simulink model "asbQuadcopters_SiFi"  (Simulink 9.1)
settings: Solver=VariableStepAuto  StartTime=0.0  StopTime=TFinal  RelTol=1e-3
values from neighbouring files (symbols this model uses):
  Controller =     [data_set.mat]
  Estimator =     [data_set.mat]
  g = 9.81    [data_set.mat]
  init =     [data_set.mat]
  rho = 1.184    [data_set.mat]
  sensorCalibrationData = [0.09 -0.06 -9.473 -0.0095 -0.0075 0.0015 101270.95 0.2]    [data_set.mat]
  Sensors =     [data_set.mat]
  States =     [data_set.mat]
  takeOffDuration = 1    [data_set.mat]
  Ts = 0.005    [data_set.mat]
  Vehicle =     [data_set.mat]
undefined symbols (not defined in the file or in its folder): DiscIntNeverNeededParam, Discrete, Earth, ft, m, s, sigbuilder_block, Time, WGS84
libraries: F_Line_block x565, simulink x39, aerolibconvert2 x4, sharedutil x3, ctrlSharedLib x3, sharedtransform x3, shared6dof x1, aerolibasang x1, aerolibtransform2 x1, aerolibnav x1, aerolibanimutils x1
(part 1 of 4)
settings Model: SuppressorTable="22 serialization::archive 11 0 6 0 0 1 8 0 0 0 0 6 0 0 1 0 44 asbQuadcopters_SiFi/Command/Live Time  Ticks 0 6 0 0 2 8 0 0 0 0 6 40 SimulinkFixedPoint:util:Overflowoccurred 0 0 0 6 0  0  0 0 0 0 8 20160523 0 0 0 10 57 55 0 1 41 Simulink:DataType:WarningOverFlowDetected 0 0 0  0  8 20160523 0 10 57 55 0 1"  LogicAnalyzerSignalOrdering=2e0c0a72-345e-4dc5-9c0e-29032ec30a1e,a96d9f9d-3ef5-4050-b6b8-b8019fd01667,c8d366ad-4d1f-40bd-a54a-09e26b883270,8941bdc4-4fa0-4569-8040-854ce7cb60c2,e7686d44-45c9-4c55-ba5d-06b91bc522a8,a75aae3c-0a7a-4dbc-8a75-97ed30805da8,7c481f21-a942-450d-9b23-3950506eae04,f4ffd508-2ff6-4be3-84ec-4b50dbf29143,1f3924a1-458c-46a2-8b2c-9c14621b8789,e4a67875-028c-4c14-9c8e-409b915de7ac,3b040215-8b3b-4fa4-83ba-2b8f885f07c0,7ff985bf-1692-4a42-b522-9402795b0a0a,96801311-fbc9-43fc-990a-89459d04cf60,3f7e7f5b-3af5-4c93-b146-0b101a8142d3,0d3d2d37-5424-425c-a4de-334d08617026,580b7cd5-bf48-4c17-856d-375ec7fff404,90f02cb4-483b-4429-aad1-b2fbf7021789,01f89b71-6786-463e-ad11-352fa7f1c28f,02989868-8137-4d3a-8960-166047eeff4b,308ffb0e-b64a-44ed-9876-4b581e92a88e,997ea37c-b9fb-41ea-9c95-cc50f5cdec72,ae01c4b6-24f8-47f4-a500-9399ba671a3d,bf52121c-d275-4d5a-9ed0-41089465bc65  Creator=DES  LastModifiedBy=dongw
settings DataIOCC: SaveFormat=Dataset
settings OptimizationCC: LifeSpan=auto
settings DebuggingCC: UnderspecifiedInitializationDetection=Simplified  MergeDetectMultiDrivingBlocksExec=error  SFUnexpectedBacktrackingDiag=error  SFNoUnconditionalDefaultTransitionDiag=error  SFExecutionAtInitializationDiag=warning
settings HardwareCC: ProdBitPerPointer=64  ProdBitPerSizeT=64  ProdBitPerPtrDiffT=64  ProdLargestAtomicFloat=Float  ProdIntDivRoundTo=Zero  ProdEndianess=LittleEndian  ProdWordSize=64  ProdHWDeviceType=Intel->x86-64 (Windows64)
settings ModelReferenceCC: PropagateSignalLabelsOutOfModel=on
settings CodeAppCC: StateflowObjectComments=off
settings GRTTargetCC: TargetLangStandard=C99 (ISO)  CombineOutputUpdateFcns=on  GRTInterface=off
settings ConfigComp: CovMetricSettings=dwe  CovHtmlReporting=off  CovSaveCumulativeToWorkspaceVar=off  CovSaveSingleToWorkspaceVar=off  CovExternalEMLEnable=on

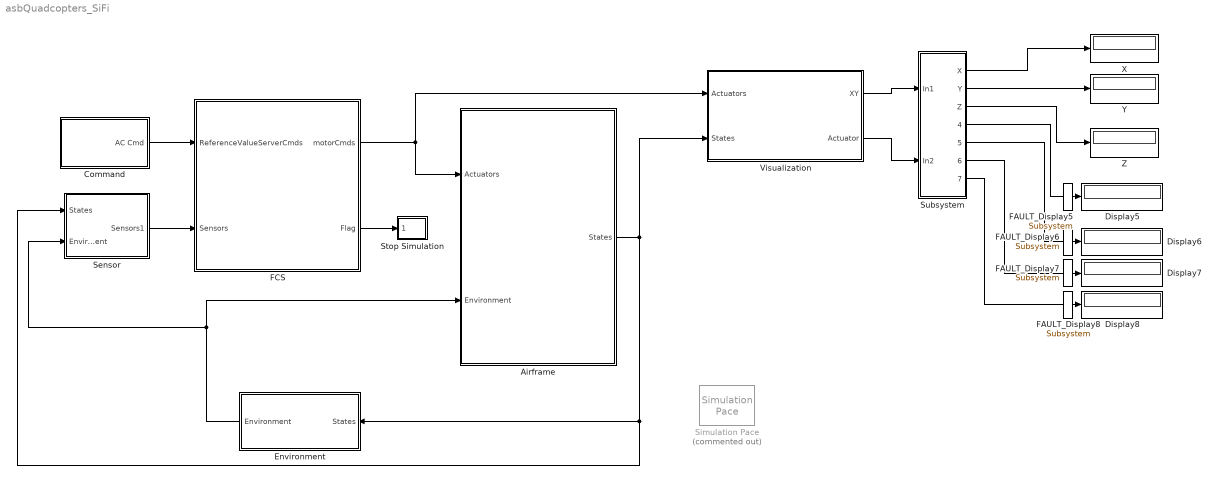
== system asbQuadcopters_SiFi ==
  Airframe : Subsystem  TreatAsAtomicUnit=on
  Command : Subsystem
  Display{5..8} (4 alike) : Display
  FAULT_Display{5..8} (4 alike) : F_Line_block/Subsystem
  Environment : Subsystem
  FCS : Subsystem
  Sensor : Subsystem
  Simulation Pace : aerolibanimutils/Simulation Pace  Commented=on  SimulationPace=1  SleepMode=MATLAB Thread  OutputPaceError=off  SampleTime=Ts
      settings: AttributesFormatString=%<SimulationPace> sec/sec
  Stop Simulation : Subsystem
  Subsystem : Subsystem
  Visualization : Subsystem
  X : Display
  Y : Display
  Z : Display
  wires:
  Command/1(AC Cmd) -> FCS/1(ReferenceValueServerCmds)
  Sensor/1(Sensors1) -> FCS/2(Sensors)
  Airframe/1(States) -> Visualization/2(States), Sensor/1(States), Environment/1(States)
  Environment/1(Environment) -> Sensor/2(Environment), Airframe/2(Environment)
  FCS/2(Flag) -> Stop Simulation/1(Flags)
  FCS/1(motorCmds) -> Visualization/1(Actuators), Airframe/1(Actuators)
  Visualization/1(XY) -> Subsystem/1(In1)
  Visualization/2(Actuator) -> Subsystem/2(In2)
  Subsystem/1(X) -> X/1
  Subsystem/2(Y) -> Y/1
  Subsystem/3(Z) -> Z/1
  Subsystem/4(Motor 1) -> Display5/1
  Subsystem/5(Motor 2) -> Display6/1
  Subsystem/6(Motor 3) -> Display7/1
  Subsystem/7(Motor 4) -> Display8/1

== system asbQuadcopters_SiFi/Airframe ==
  Actuators : Inport
  Environment : Inport  Port=2
  6DOF (Quaternion) : shared6dof/6DOF (Euler Angles)  units=Metric (MKS)  mtype=Fixed  rep=Euler Angles  xme_0=init.posNED  Vm_0=init.vb  eul_0=init.euler  pm_0=init.angRates  mass_0=Vehicle.Airframe.mass  mass_e=0.5  mass_f=2.0  inertia=Vehicle.Airframe.inertia  inertia_e=eye(3)  inertia_f=2*eye(3)  k_quat=Vehicle.SixDOF.quatGain  vre_flag=on  abi_flag=on  aMode=aMode
      settings: SourceProductBaseCode=AE
  FAULT_6DOF (Quaternion) : F_Line_block/Subsystem
  FAULT_6DOF (Quaternion)_2 : F_Line_block/Subsystem
  AC model : Subsystem
  Bus setup : Subsystem
  Position on Earth : Subsystem  Priority=1  TreatAsAtomicUnit=on
  Terminator : Terminator
  FAULT_Terminator : F_Line_block/Subsystem
  States : Outport
  FAULT_States : F_Line_block/Subsystem
  wires:
  Actuators/1 -> AC model/1(Actuators)
  Environment/1 -> AC model/2(Environment)
  AC model/1(F_cg) -> FAULT_6DOF (Quaternion)/1
  FAULT_6DOF (Quaternion)/1 -> 6DOF (Quaternion)/1
  AC model/2(M_cg) -> FAULT_6DOF (Quaternion)_2/1
  FAULT_6DOF (Quaternion)_2/1 -> 6DOF (Quaternion)/2
  6DOF (Quaternion)/1 -> Bus setup/2(V_ned)
  6DOF (Quaternion)/2 -> Position on Earth/1(Xe), Bus setup/3(X_ned)
  6DOF (Quaternion)/3 -> Bus setup/4(Euler)
  6DOF (Quaternion)/6 -> AC model/5(w_b), Bus setup/7(Omega_b)
  6DOF (Quaternion)/7 -> Bus setup/8(dOmega_b)
  6DOF (Quaternion)/9 -> Bus setup/9(Accel_b)
  Bus setup/1(States) -> FAULT_States/1
  ?FAULT_Product7/1 -> ?Product7/1
  ?FAULT_Product6_2/1 -> ?Product6/2
  ?FAULT_Selector2/1 -> ?Selector2/1
  FAULT_States/1 -> States/1
  Position on Earth/1(LLA) -> Bus setup/1(LLA)
  6DOF (Quaternion)/5 -> AC model/4(V_b), Bus setup/6(V_b)
  6DOF (Quaternion)/4 -> AC model/3(DCM_be), Bus setup/5(DCM_be)
  6DOF (Quaternion)/8 -> FAULT_Terminator/1
  ?FAULT_Product7/1 -> ?Product7/1
  ?FAULT_Product6_2/1 -> ?Product6/2
  ?FAULT_Selector2/1 -> ?Selector2/1
  FAULT_Terminator/1 -> Terminator/1

== system asbQuadcopters_SiFi/Command ==
  Bus Creator : BusCreator  Inputs=5  OutDataTypeStr=Bus: CommandBus  NonVirtualBus=on
  Clock : Clock
  FAULT_Clock : F_Line_block/Subsystem
  Compare To Constant : simulink/Logic and Bit Operations/Compare To Constant  relop=<  const=takeOffDuration  OutDataTypeStr=boolean
  FAULT_Compare To Constant : F_Line_block/Subsystem
  Compare To Zero : simulink/Logic and Bit Operations/Compare To Zero  relop===  OutDataTypeStr=boolean
  FAULT_Compare To Zero : F_Line_block/Subsystem
  Compare To Zero1 : simulink/Logic and Bit Operations/Compare To Zero  relop===  OutDataTypeStr=boolean
  FAULT_Compare To Zero1 : F_Line_block/Subsystem
  Data Type Conversion1 : DataTypeConversion  OutDataTypeStr=single
  FAULT_Data Type Conversion1 : F_Line_block/Subsystem
  Data Type Conversion3 : DataTypeConversion  OutDataTypeStr=single
  FAULT_Data Type Conversion3 : F_Line_block/Subsystem
  Live Time  Ticks : simulink/Sources/Counter Free-Running  NumBits=32  tsamp=Ts
  FAULT_Live Time  Ticks : F_Line_block/Subsystem
  Logical Operator : Logic  AllPortsSameDT=off  OutDataTypeStr=boolean
  FAULT_Logical Operator : F_Line_block/Subsystem
  FAULT_Logical Operator_2 : F_Line_block/Subsystem
  Mux : Mux  Inputs=3
  FAULT_Mux : F_Line_block/Subsystem
  FAULT_Mux_2 : F_Line_block/Subsystem
  FAULT_Mux_3 : F_Line_block/Subsystem
  Mux1 : Mux  Inputs=3
  FAULT_Mux1 : F_Line_block/Subsystem
  FAULT_Mux1_2 : F_Line_block/Subsystem
  FAULT_Mux1_3 : F_Line_block/Subsystem
  Position/Attitude Reference : Subsystem  Tag=STV Subsys  LoadFcn=sigbuilder_block('load');  StartFcn=sigbuilder_block('start');  StopFcn=sigbuilder_block('stop');  ClipboardFcn=sigbuilder_block('clipboard');  mask(Sigbuilder block){tuvar=[0:10]}
      mask help: Simulink:masks:SigbuilderBlock_MD
      mask init:
      | if ~strcmp(get_param(bdroot(gcbh),'SimulationStatus'),'stopped') tuvar = sigbuilder_block('maskInit'); end
      settings: CopyFcn=sigbuilder_block('copy');  DeleteFcn=sigbuilder_block('delete');  ModelCloseFcn=sigbuilder_block('modelClose');  PreSaveFcn=sigbuilder_block('preSave');  PauseFcn=sigbuilder_block('pause');  ContinueFcn=sigbuilder_block('continue');  NameChangeFcn=sigbuilder_block('namechange');  OpenFcn=sigbuilder_block('open',[0 30 1440 721.5 ]);  CloseFcn=sigbuilder_block('close');
      mask Display: plot(0, 0, 100, 100,[2, 2, 32, 32, 2], [68, 8, 8, 68, 68],[32, 2], [38, 38], [32, 19, 2],[53, 60, 44], [32, 17, 17, 2],[16, 16, 31, 31]);txt = getActiveGroup(gcbh);text(2, 100, txt,'verticalAlignment', 'top');
  Rate Transition{1..4} (4 alike) : RateTransition  OutPortSampleTime=Ts
  FAULT_Rate Transition{1..4} (4 alike) : F_Line_block/Subsystem
  AC Cmd : Outport  OutDataTypeStr=Bus: CommandBus
  FAULT_AC Cmd : F_Line_block/Subsystem
  wires:
  Bus Creator/1 -> FAULT_AC Cmd/1
  FAULT_AC Cmd/1 -> AC Cmd/1
  Position/Attitude Reference/3(Z) -> FAULT_Mux1_3/1
  FAULT_Mux1_3/1 -> Mux1/3
  Live Time  Ticks/1 -> Bus Creator/5  "live_time_ticks"
  Position/Attitude Reference/6(Roll) -> FAULT_Compare To Zero/1, FAULT_Mux_3/1  "roll_cmd"
  FAULT_Compare To Zero/1 -> Compare To Zero/1
  FAULT_Mux_3/1 -> Mux/3
  Position/Attitude Reference/5(Pitch) -> FAULT_Mux_2/1, FAULT_Compare To Zero1/1  "pitch_cmd"
  FAULT_Mux_2/1 -> Mux/2
  FAULT_Compare To Zero1/1 -> Compare To Zero1/1
  Compare To Zero1/1 -> FAULT_Logical Operator_2/1
  FAULT_Logical Operator_2/1 -> Logical Operator/2
  Rate Transition4/1 -> Bus Creator/1  "controlModePosVSOrient"
  Position/Attitude Reference/2(Y) -> FAULT_Mux1_2/1
  FAULT_Mux1_2/1 -> Mux1/2
  Rate Transition3/1 -> Bus Creator/3  "takeoff_flag"
  Position/Attitude Reference/4(Yaw) -> FAULT_Mux/1  "yaw_cmd"
  FAULT_Mux/1 -> Mux/1
  Data Type Conversion1/1 -> FAULT_Rate Transition2/1
  FAULT_Rate Transition2/1 -> Rate Transition2/1
  Compare To Zero/1 -> FAULT_Logical Operator/1
  FAULT_Logical Operator/1 -> Logical Operator/1
  Logical Operator/1 -> FAULT_Rate Transition4/1
  FAULT_Rate Transition4/1 -> Rate Transition4/1
  Mux1/1 -> FAULT_Data Type Conversion1/1
  FAULT_Data Type Conversion1/1 -> Data Type Conversion1/1
  Mux/1 -> FAULT_Data Type Conversion3/1
  FAULT_Data Type Conversion3/1 -> Data Type Conversion3/1
  Rate Transition2/1 -> Bus Creator/2  "pos_ref"
  Data Type Conversion3/1 -> FAULT_Rate Transition1/1
  FAULT_Rate Transition1/1 -> Rate Transition1/1
  Compare To Constant/1 -> FAULT_Rate Transition3/1
  FAULT_Rate Transition3/1 -> Rate Transition3/1
  Clock/1 -> FAULT_Compare To Constant/1
  FAULT_Compare To Constant/1 -> Compare To Constant/1
  Rate Transition1/1 -> Bus Creator/4  "orient_ref"
  Position/Attitude Reference/1(X) -> FAULT_Mux1/1
  FAULT_Mux1/1 -> Mux1/1

== system asbQuadcopters_SiFi/Environment ==
  States : Inport  OutDataTypeStr=Bus: StatesBus
  Air Density : Constant  Value=rho
  Air Temp : Constant  Value=273+15
  Bus Creator : BusCreator  Inputs=3  OutDataTypeStr=Bus: EnvironmentBus  NonVirtualBus=on
  Bus Creator1 : BusCreator  Inputs=4  OutDataTypeStr=Bus: AtmosphereBus  NonVirtualBus=on
  Gravity : Constant  Value=[0 0 g]
  Magnetic Field : Constant  Value=[0 0 0]
  Pressure : Constant  Value=101.3e3
  Speed of Sound : Constant  Value=340
  Terminator : Terminator
  FAULT_Terminator : F_Line_block/Subsystem
  Environment : Outport  OutDataTypeStr=Bus: EnvironmentBus
  FAULT_Environment : F_Line_block/Subsystem
  wires:
  Speed of Sound/1 -> Bus Creator1/2  "speed_sound"
  Air Density/1 -> Bus Creator1/4  "air_density"
  Magnetic Field/1 -> Bus Creator/3  "MagneticField_ned"
  Bus Creator/1 -> FAULT_Environment/1
  FAULT_Environment/1 -> Environment/1
  Gravity/1 -> Bus Creator/1  "Gravity_ned"
  Bus Creator1/1 -> Bus Creator/2  "AtmosphereBus"
  States/1 -> FAULT_Terminator/1
  FAULT_Terminator/1 -> Terminator/1
  Air Temp/1 -> Bus Creator1/1  "air_temp"
  Pressure/1 -> Bus Creator1/3  "pressure"

== system asbQuadcopters_SiFi/FCS ==
  note: Derived from the work by Sertac
      | Karaman and Fabian Riether
  ReferenceValueServerCmds : Inport  OutDataTypeStr=Bus: CommandBus
  Sensors : Inport  Port=2  OutDataTypeStr=Bus: SensorsBus  BusOutputAsStruct=on
  Bus Selector : BusSelector  OutputSignals=controlModePosVSOrient
  Bus Selector1 : BusSelector  OutputSignals=usePosVIS_flag,opticalFlow_data,posVIS_data
  Bus Selector2 : BusSelector  OutputSignals=HAL_acc_SI,HAL_gyro_SI,HAL_ultrasound_SI,HAL_pressure_SI,HAL_vbat_SI
  Bus Selector3 : BusSelector  OutputSignals=HALSensors
  Bus Selector4 : BusSelector  OutputSignals=VisionSensors,SensorCalibration
  Crash Predictor Flags : Subsystem
  Logging : Subsystem  TreatAsAtomicUnit=on
      settings: RTWFcnNameOpts=Use subsystem name
  ReferenceValueServerCmds_1 : InportShadow  OutDataTypeStr=Bus: CommandBus
  Sensors_1 : InportShadow  Port=2  OutDataTypeStr=Bus: SensorsBus  BusOutputAsStruct=on
  Sensors_2 : InportShadow  Port=2  OutDataTypeStr=Bus: SensorsBus  BusOutputAsStruct=on
  State Estimator : Subsystem
  controller : Subsystem
  sensordata_group : Subsystem
  motorCmds : Outport
  Flag : Outport  Port=2
  wires:
  Bus Selector4/2 -> State Estimator/6(sensorCalibration_datin)  "<SensorCalibration>"
  Bus Selector3/1 -> Bus Selector2/1  "<HALSensors>"
  Bus Selector1/3 -> State Estimator/5(posVIS_datin)  "<posVIS_data>"
  Bus Selector/1 -> State Estimator/1(controlModePosVSOrient_flagin)  "<controlModePosVSOrient>"
  Bus Selector2/1 -> sensordata_group/1(HAL_acc_SI)  "<HAL_acc_SI>"
  State Estimator/1(states_estim) -> controller/2(states_estim), Crash Predictor Flags/1(states_estim), Logging/3(states_estim)
  controller/1(motors_refout) -> motorCmds/1, Logging/1(motorCmds)
  Bus Selector2/4 -> sensordata_group/4(HAL_pressure_SI)  "<HAL_pressure_SI>"
  Bus Selector1/1 -> State Estimator/3(usePosVIS_flagin)  "<usePosVIS_flag>"
  sensordata_group/1(sensordata_datin) -> State Estimator/2(sensor_data_in), Logging/6(sensordata_datin)
  Bus Selector1/2 -> State Estimator/4(opticalFlow_datin)  "<opticalFlow_data>"
  ReferenceValueServerCmds/1 -> controller/1(ReferenceValueServerBus), Bus Selector/1
  controller/2(pose_refout) -> Logging/2(posRef)
  Bus Selector4/1 -> Bus Selector1/1  "<VisionSensors>"
  Sensors_1/1 -> Crash Predictor Flags/2(Sensors), Bus Selector4/1
  Bus Selector2/2 -> sensordata_group/2(HAL_gyro_SI)  "<HAL_gyro_SI>"
  Bus Selector2/3 -> sensordata_group/3(HAL_ultrasound_SI)  "<HAL_ultrasound_SI>"
  Sensors/1 -> Bus Selector3/1
  Crash Predictor Flags/1(Flag) -> Flag/1
  Sensors_2/1 -> Logging/5(Sensors)
  Bus Selector2/5 -> sensordata_group/5(HAL_vbat_SI)  "<HAL_vbat_SI>"
  ReferenceValueServerCmds_1/1 -> Logging/4(ReferenceValueServerBus)

== system asbQuadcopters_SiFi/Sensor ==
  States : Inport  OutDataTypeStr=Bus: StatesBus
  Environment : Inport  Port=2  OutDataTypeStr=Bus: EnvironmentBus
  Bus Creator1 : BusCreator  Inputs=3  OutDataTypeStr=Bus: SensorsBus  NonVirtualBus=on
  Bus Creator2 : BusCreator  Inputs=3  OutDataTypeStr=Bus: extraSensorData_t  NonVirtualBus=on
  Constant : Constant  Value=sensorCalibrationData  OutDataTypeStr=single
  Memory1 : Memory  InitialCondition=States  InheritSampleTime=on
  Sensor System : Subsystem
  _DUMMY_FLAG_usePosVIS : Constant  Value=Sensors.dummy.usePosVISFlag  OutDataTypeStr=single  SampleTime=Ts
  _DUMMY_posVIS : Constant  Value=Sensors.dummy.posVISNoVisionAvail  OutDataTypeStr=single  SampleTime=Ts
  Sensors1 : Outport  OutDataTypeStr=Bus: SensorsBus
  wires:
  Memory1/1 -> Sensor System/1(States)
  Bus Creator2/1 -> Bus Creator1/1  "VisionSensors"
  Sensor System/1(opticalFlow_data) -> Bus Creator2/1  "opticalFlow_data"
  Environment/1 -> Sensor System/2(Environment)
  Sensor System/2(sensordata_data) -> Bus Creator1/2  "HALSensors"
  Bus Creator1/1 -> Sensors1/1
  States/1 -> Memory1/1
  _DUMMY_posVIS/1 -> Bus Creator2/2  "posVIS_data"
  Constant/1 -> Bus Creator1/3  "SensorCalibration"
  _DUMMY_FLAG_usePosVIS/1 -> Bus Creator2/3  "usePosVIS_flag"

== system asbQuadcopters_SiFi/Stop Simulation ==
  Flags : Inport  OutDataTypeStr=uint8
  Compare To Zero : simulink/Logic and Bit Operations/Compare To Zero  relop=>  OutDataTypeStr=boolean
  Flag has been triggered : Assertion
  Logical Operator : Logic  Operator=NOT  AllPortsSameDT=off  OutDataTypeStr=boolean
  wires:
  Flags/1 -> Compare To Zero/1
  Logical Operator/1 -> Flag has been triggered/1
  Compare To Zero/1 -> Logical Operator/1

== system asbQuadcopters_SiFi/Subsystem ==
  In1 : Inport
  In2 : Inport  Port=2
  Constant : Constant  Value=57
  Constant1 : Constant  Value=95
  Demux : Demux  Outputs=3
  Demux1 : Demux
  Minus : Sum  Inputs=+-
  Minus1 : Sum  Inputs=+-
  X : Outport
  Y : Outport  Port=2
  Z : Outport  Port=3
  Motor 1 : Outport  Port=4
  Motor 2 : Outport  Port=5
  Motor 3 : Outport  Port=6
  Motor 4 : Outport  Port=7
  wires:
  Demux1/3 -> Motor 3/1
  Constant1/1 -> Minus1/2
  Minus1/1 -> Y/1
  Demux1/4 -> Motor 4/1
  Demux1/2 -> Motor 2/1
  Demux/1 -> Minus/1
  Demux/2 -> Minus1/1
  Constant/1 -> Minus/2
  Demux1/1 -> Motor 1/1
  Minus/1 -> X/1
  In2/1 -> Demux1/1
  Demux/3 -> Z/1
  In1/1 -> Demux/1

== system asbQuadcopters_SiFi/Visualization ==
  Actuators : Inport
  States : Inport  Port=2
  Extract Flight Instruments : Subsystem
  XY : Outport
  Actuator : Outport  Port=2
  wires:
  Actuators/1 -> Extract Flight Instruments/1(Actuators)
  States/1 -> Extract Flight Instruments/2(States)
  Extract Flight Instruments/1(XY) -> XY/1
  Extract Flight Instruments/2(Actuator) -> Actuator/1

== system asbQuadcopters_SiFi/Airframe/AC model ==
  Actuators : Inport
  Environment : Inport  Port=2
  DCM_be : Inport  Port=3
  V_b : Inport  Port=4  Unit=m/s
  w_b : Inport  Port=5  Unit=rad/s
  Applied Force Calculation : Subsystem
  Bus Selector : BusSelector  OutputSignals=Gravity_ned,AtmosphereBus.air_density
  Drag Calculation : Subsystem
  Gravity Force Calculation : Subsystem
  Motor Forces and Torques : Subsystem
  F_cg : Outport  Unit=N
  FAULT_F_cg : F_Line_block/Subsystem
  M_cg : Outport  Port=2  Unit=N*m
  FAULT_M_cg : F_Line_block/Subsystem
  wires:
  Applied Force Calculation/1(External Forces) -> FAULT_F_cg/1
  FAULT_F_cg/1 -> F_cg/1
  Motor Forces and Torques/2(Motor Torques) -> FAULT_M_cg/1
  FAULT_M_cg/1 -> M_cg/1
  Motor Forces and Torques/1(Motor Forces) -> Applied Force Calculation/3(Motor Forces)
  Bus Selector/1 -> Gravity Force Calculation/2(gravity)  "<Gravity_ned>"
  Gravity Force Calculation/1(gravity force) -> Applied Force Calculation/1(gravity force)
  Environment/1 -> Bus Selector/1
  Bus Selector/2 -> Motor Forces and Torques/2(Density), Drag Calculation/1(Density)  "<air_density>"
  DCM_be/1 -> Gravity Force Calculation/1(DCMbe)
  V_b/1 -> Motor Forces and Torques/1(Vb), Drag Calculation/2(Vb)
  Drag Calculation/1(Drag) -> Applied Force Calculation/2(Aerodynamic Forces)
  Actuators/1 -> Motor Forces and Torques/4(Motor  Commands)
  w_b/1 -> Motor Forces and Torques/3(pqr)

== system asbQuadcopters_SiFi/Airframe/Bus setup ==
  LLA : Inport  PortDimensions=3
  V_ned : Inport  Port=2  Unit=m/second  PortDimensions=3
  X_ned : Inport  Port=3  Unit=m  PortDimensions=3
  Euler : Inport  Port=4  Unit=rad  PortDimensions=3
  DCM_be : Inport  Port=5  PortDimensions=[3 3]
  V_b : Inport  Port=6  Unit=m/s  PortDimensions=3
  Omega_b : Inport  Port=7  Unit=rad/s  PortDimensions=3
  dOmega_b : Inport  Port=8  Unit=rad/s^2  PortDimensions=3
  Accel_b : Inport  Port=9  Unit=m/s^2  PortDimensions=3
  Bus Creator5 : BusCreator  Inputs=9  OutDataTypeStr=Bus: StatesBus  NonVirtualBus=on
  States : Outport
  FAULT_States : F_Line_block/Subsystem
  wires:
  Bus Creator5/1 -> FAULT_States/1
  ?FAULT_Product7/1 -> ?Product7/1
  ?FAULT_Product6_2/1 -> ?Product6/2
  ?FAULT_Selector2/1 -> ?Selector2/1
  FAULT_States/1 -> States/1
  V_b/1 -> Bus Creator5/1  "V_body"
  Omega_b/1 -> Bus Creator5/2  "Omega_body"
  Euler/1 -> Bus Creator5/3  "Euler"
  X_ned/1 -> Bus Creator5/7  "X_ned"
  Accel_b/1 -> Bus Creator5/4  "Accel_body"
  LLA/1 -> Bus Creator5/8  "LLA"
  dOmega_b/1 -> Bus Creator5/5  "dOmega_body"
  DCM_be/1 -> Bus Creator5/9  "DCM_be"
  V_ned/1 -> Bus Creator5/6  "V_ned"

== system asbQuadcopters_SiFi/Airframe/Position on Earth ==
  Xe : Inport  Unit=m
  Flat Earth to LLA : aerolibtransform2/Flat Earth to LLA  units=Metric (MKS)  ptype=Earth (WGS84)  F=1/298.257223563  R=6378137  LL0=init.posLLA(1:2)  psi=Vehicle.PositionOnEarth.FlatEarthToLLA.xAxis
  FAULT_Flat Earth to LLA : F_Line_block/Subsystem
  FAULT_Flat Earth to LLA_2 : F_Line_block/Subsystem
  Mux : Mux  Inputs=2
  FAULT_Mux : F_Line_block/Subsystem
  FAULT_Mux_2 : F_Line_block/Subsystem
  href : Constant  Value=Vehicle.PositionOnEarth.href
  LLA : Outport
  FAULT_LLA : F_Line_block/Subsystem
  wires:
  Mux/1 -> FAULT_LLA/1
  FAULT_LLA/1 -> LLA/1
  Xe/1 -> FAULT_Flat Earth to LLA/1
  FAULT_Flat Earth to LLA/1 -> Flat Earth to LLA/1
  Flat Earth to LLA/1 -> FAULT_Mux/1
  FAULT_Mux/1 -> Mux/1
  Flat Earth to LLA/2 -> FAULT_Mux_2/1
  FAULT_Mux_2/1 -> Mux/2
  href/1 -> FAULT_Flat Earth to LLA_2/1
  FAULT_Flat Earth to LLA_2/1 -> Flat Earth to LLA/2

== system asbQuadcopters_SiFi/Command/Position/Attitude Reference ==
  Demux : Demux  Tag=STV Demux  Outputs=6
  FAULT_Demux : F_Line_block/Subsystem
  FromWs : FromWorkspace  Tag=STV FromWs  VariableName=tuvar  SampleTime=0  SigBuilderData=DataTag0  VnvData=DataTag1
      SigBuilderData=|
      | common.afterFinalStr = 'Extrapolate'
      | common.sampleTime = 0
      | dataSet.timeRange = [0 100]
      | dataSet.name = 'Group 1'
      | sbobj.Groups.Name = 'Group 1'
      | sbobj.Groups.Signals(1).Name = 'X'
      | sbobj.Groups.Signals(1).XData = [0 4 6 100]
      | sbobj.Groups.Signals(1).YData = [0 0 0 0]
      | sbobj.Groups.Signals(2).Name = 'Y'
      | sbobj.Groups.Signals(2).XData = [0 4 6 100]
      | sbobj.Groups.Signals(2).YData = [0 0 0 0]
      | sbobj.Groups.Signals(3).Name = 'Z'
      | sbobj.Groups.Signals(3).XData = [0 1 1 6 100]
      | sbobj.Groups.Signals(3).YData = [0 0 -1.8 -1.8 -1.8]
      | sbobj.Groups.Signals(4).Name = 'Yaw'
      | sbobj.Groups.Signals(4).XData = [0 4 6 100]
      | sbobj.Groups.Signals(4).YData = [0 0 0 0]
      | sbobj.Groups.Signals(5).Name = 'Pitch'
      | sbobj.Groups.Signals(5).XData = [0 4 6 100]
      | sbobj.Groups.Signals(5).YData = [0 0 0 0]
      | sbobj.Groups.Signals(6).Name = 'Roll'
      | sbobj.Groups.Signals(6).XData = [0 4 6 100]
      | sbobj.Groups.Signals(6).YData = [0 0 0 0]
      | sbobj.Groups.TimeRange = [0 100]
  X : Outport  Tag=STV Outport
  FAULT_X : F_Line_block/Subsystem
  Y : Outport  Tag=STV Outport  Port=2
  FAULT_Y : F_Line_block/Subsystem
  Z : Outport  Tag=STV Outport  Port=3
  FAULT_Z : F_Line_block/Subsystem
  Yaw : Outport  Tag=STV Outport  Port=4
  FAULT_Yaw : F_Line_block/Subsystem
  Pitch : Outport  Tag=STV Outport  Port=5
  FAULT_Pitch : F_Line_block/Subsystem
  Roll : Outport  Tag=STV Outport  Port=6
  FAULT_Roll : F_Line_block/Subsystem
  wires:
  Demux/1 -> FAULT_X/1
  FAULT_X/1 -> X/1
  FromWs/1 -> FAULT_Demux/1
  FAULT_Demux/1 -> Demux/1
  Demux/2 -> FAULT_Y/1
  FAULT_Y/1 -> Y/1
  Demux/3 -> FAULT_Z/1
  FAULT_Z/1 -> Z/1
  Demux/4 -> FAULT_Yaw/1
  FAULT_Yaw/1 -> Yaw/1
  Demux/5 -> FAULT_Pitch/1
  FAULT_Pitch/1 -> Pitch/1
  Demux/6 -> FAULT_Roll/1
  FAULT_Roll/1 -> Roll/1

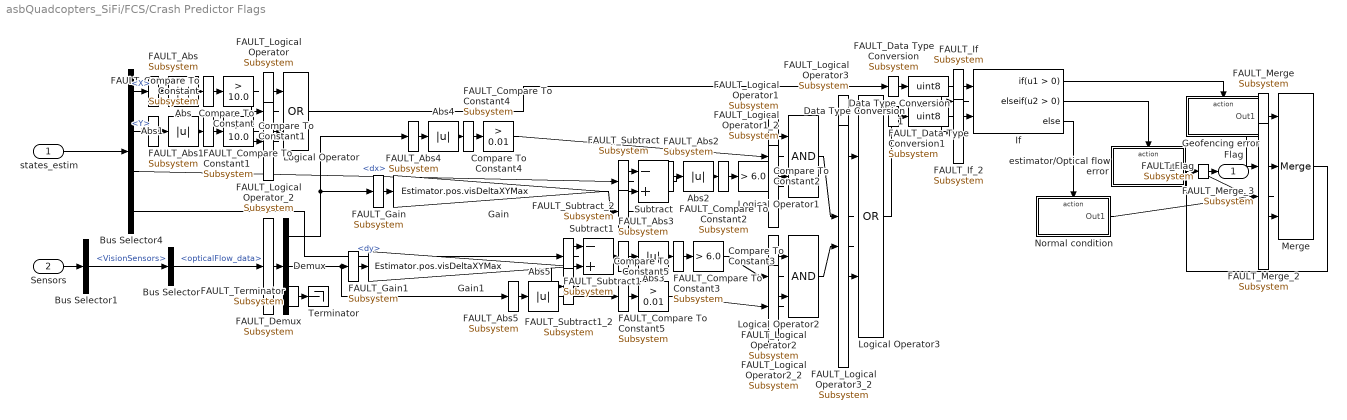
== system asbQuadcopters_SiFi/FCS/Crash Predictor Flags ==
  states_estim : Inport
  Sensors : Inport  Port=2
  Abs{,1..5} (6 alike) : Abs
  FAULT_Abs{,1..5} (6 alike) : F_Line_block/Subsystem
  Bus Selector : BusSelector  OutputSignals=opticalFlow_data
  Bus Selector1 : BusSelector  OutputSignals=VisionSensors
  Bus Selector4 : BusSelector  OutputSignals=X,Y,dx,dy
  Compare To Constant : simulink/Logic and Bit Operations/Compare To Constant  relop=>  const=10.0  OutDataTypeStr=boolean
  FAULT_Compare To Constant{,1..5} (6 alike) : F_Line_block/Subsystem
  Compare To Constant1 : simulink/Logic and Bit Operations/Compare To Constant  relop=>  const=10.0  OutDataTypeStr=boolean
  Compare To Constant2 : simulink/Logic and Bit Operations/Compare To Constant  relop=>  const=6.0  OutDataTypeStr=boolean
  Compare To Constant3 : simulink/Logic and Bit Operations/Compare To Constant  relop=>  const=6.0  OutDataTypeStr=boolean
  Compare To Constant4 : simulink/Logic and Bit Operations/Compare To Constant  relop=>  const=0.01  OutDataTypeStr=boolean
  Compare To Constant5 : simulink/Logic and Bit Operations/Compare To Constant  relop=>  const=0.01  OutDataTypeStr=boolean
  Data Type Conversion : DataTypeConversion  OutDataTypeStr=uint8  RndMeth=Nearest
  FAULT_Data Type Conversion : F_Line_block/Subsystem
  Data Type Conversion1 : DataTypeConversion  OutDataTypeStr=uint8  RndMeth=Nearest
  FAULT_Data Type Conversion1 : F_Line_block/Subsystem
  Demux : Demux  Outputs=3
  FAULT_Demux : F_Line_block/Subsystem
  Gain : Gain  Gain=Estimator.pos.visDeltaXYMax
  FAULT_Gain : F_Line_block/Subsystem
  Gain1 : Gain  Gain=Estimator.pos.visDeltaXYMax
  FAULT_Gain1 : F_Line_block/Subsystem
  Geofencing error : Subsystem  TreatAsAtomicUnit=on
  If : If  NumInputs=2  ElseIfExpressions=u2 > 0
  FAULT_If : F_Line_block/Subsystem
  FAULT_If_2 : F_Line_block/Subsystem
  Logical Operator : Logic  Operator=OR  AllPortsSameDT=off
  FAULT_Logical Operator{,1..3} (4 alike) : F_Line_block/Subsystem
  FAULT_Logical Operator_2 : F_Line_block/Subsystem
  Logical Operator1 : Logic  AllPortsSameDT=off  OutDataTypeStr=boolean
  FAULT_Logical Operator1_2 : F_Line_block/Subsystem
  Logical Operator2 : Logic  AllPortsSameDT=off  OutDataTypeStr=boolean
  FAULT_Logical Operator2_2 : F_Line_block/Subsystem
  Logical Operator3 : Logic  Operator=OR  AllPortsSameDT=off
  FAULT_Logical Operator3_2 : F_Line_block/Subsystem
  Merge : Merge  Inputs=3  InitialOutput=0
  FAULT_Merge : F_Line_block/Subsystem
  FAULT_Merge_2 : F_Line_block/Subsystem
  FAULT_Merge_3 : F_Line_block/Subsystem
  Normal condition : Subsystem  TreatAsAtomicUnit=on
  Subtract : Sum  Inputs=-+
  FAULT_Subtract : F_Line_block/Subsystem
  FAULT_Subtract_2 : F_Line_block/Subsystem
  Subtract1 : Sum  Inputs=-+
  FAULT_Subtract1 : F_Line_block/Subsystem
  FAULT_Subtract1_2 : F_Line_block/Subsystem
  Terminator : Terminator
  FAULT_Terminator : F_Line_block/Subsystem
  estimator/Optical flow error : Subsystem  TreatAsAtomicUnit=on
  Flag : Outport
  FAULT_Flag : F_Line_block/Subsystem
  wires:
  Bus Selector4/1 -> FAULT_Abs/1  "<X>"
  FAULT_Abs/1 -> Abs/1
  states_estim/1 -> Bus Selector4/1
  Bus Selector4/2 -> FAULT_Abs1/1  "<Y>"
  FAULT_Abs1/1 -> Abs1/1
  Compare To Constant/1 -> FAULT_Logical Operator/1
  FAULT_Logical Operator/1 -> Logical Operator/1
  Compare To Constant1/1 -> FAULT_Logical Operator_2/1
  FAULT_Logical Operator_2/1 -> Logical Operator/2
  Abs/1 -> FAULT_Compare To Constant/1
  FAULT_Compare To Constant/1 -> Compare To Constant/1
  Abs1/1 -> FAULT_Compare To Constant1/1
  FAULT_Compare To Constant1/1 -> Compare To Constant1/1
  Logical Operator/1 -> FAULT_Data Type Conversion/1
  FAULT_Data Type Conversion/1 -> Data Type Conversion/1
  Bus Selector/1 -> FAULT_Demux/1  "<opticalFlow_data>"
  FAULT_Demux/1 -> Demux/1
  Demux/1 -> FAULT_Abs4/1, FAULT_Gain/1
  FAULT_Abs4/1 -> Abs4/1
  FAULT_Gain/1 -> Gain/1
  Demux/2 -> FAULT_Gain1/1, FAULT_Abs5/1
  FAULT_Gain1/1 -> Gain1/1
  FAULT_Abs5/1 -> Abs5/1
  Bus Selector4/3 -> FAULT_Subtract/1  "<dx>"
  FAULT_Subtract/1 -> Subtract/1
  Subtract/1 -> FAULT_Abs2/1
  FAULT_Abs2/1 -> Abs2/1
  Subtract1/1 -> FAULT_Abs3/1
  FAULT_Abs3/1 -> Abs3/1
  Abs2/1 -> FAULT_Compare To Constant2/1
  FAULT_Compare To Constant2/1 -> Compare To Constant2/1
  Abs3/1 -> FAULT_Compare To Constant3/1
  FAULT_Compare To Constant3/1 -> Compare To Constant3/1
  Compare To Constant5/1 -> FAULT_Logical Operator2_2/1
  FAULT_Logical Operator2_2/1 -> Logical Operator2/2
  Abs4/1 -> FAULT_Compare To Constant4/1
  FAULT_Compare To Constant4/1 -> Compare To Constant4/1
  Abs5/1 -> FAULT_Compare To Constant5/1
  FAULT_Compare To Constant5/1 -> Compare To Constant5/1
  Compare To Constant3/1 -> FAULT_Logical Operator2/1
  FAULT_Logical Operator2/1 -> Logical Operator2/1
  Logical Operator1/1 -> FAULT_Logical Operator3/1
  FAULT_Logical Operator3/1 -> Logical Operator3/1
  Logical Operator2/1 -> FAULT_Logical Operator3_2/1
  FAULT_Logical Operator3_2/1 -> Logical Operator3/2
  Logical Operator3/1 -> FAULT_Data Type Conversion1/1
  FAULT_Data Type Conversion1/1 -> Data Type Conversion1/1
  Demux/3 -> FAULT_Terminator/1
  FAULT_Terminator/1 -> Terminator/1
  Gain/1 -> FAULT_Subtract_2/1
  FAULT_Subtract_2/1 -> Subtract/2
  Bus Selector4/4 -> FAULT_Subtract1/1  "<dy>"
  FAULT_Subtract1/1 -> Subtract1/1
  Gain1/1 -> FAULT_Subtract1_2/1
  FAULT_Subtract1_2/1 -> Subtract1/2
  Compare To Constant4/1 -> FAULT_Logical Operator1/1
  FAULT_Logical Operator1/1 -> Logical Operator1/1
  Compare To Constant2/1 -> FAULT_Logical Operator1_2/1
  FAULT_Logical Operator1_2/1 -> Logical Operator1/2
  Sensors/1 -> Bus Selector1/1
  Bus Selector1/1 -> Bus Selector/1  "<VisionSensors>"
  Merge/1 -> FAULT_Flag/1
  FAULT_Flag/1 -> Flag/1
  If/1 -> Geofencing error/Action
  If/2 -> estimator/Optical flow error/Action
  If/3 -> Normal condition/Action
  Geofencing error/1(Out1) -> FAULT_Merge/1
  FAULT_Merge/1 -> Merge/1
  estimator/Optical flow error/1(Out1) -> FAULT_Merge_2/1
  FAULT_Merge_2/1 -> Merge/2
  Normal condition/1(Out1) -> FAULT_Merge_3/1
  FAULT_Merge_3/1 -> Merge/3
  Data Type Conversion/1 -> FAULT_If/1
  FAULT_If/1 -> If/1
  Data Type Conversion1/1 -> FAULT_If_2/1
  FAULT_If_2/1 -> If/2

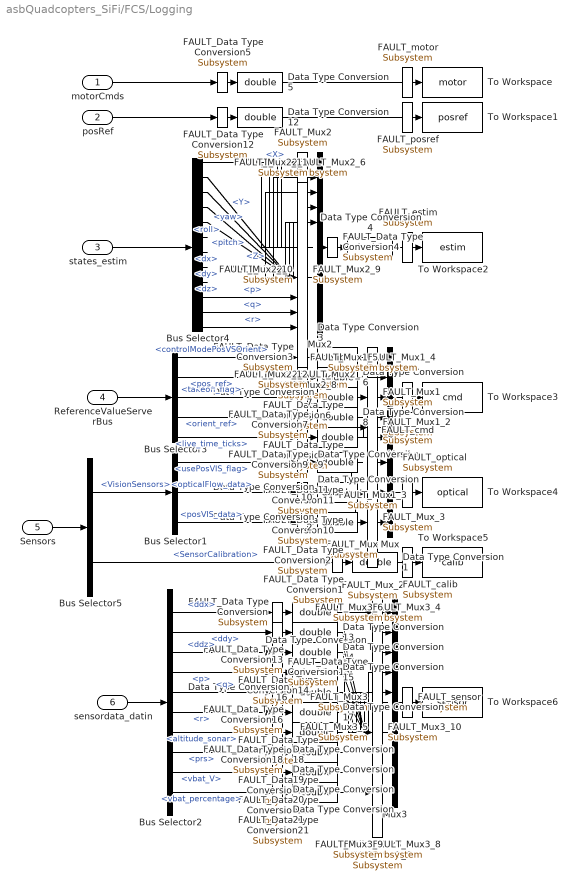
== system asbQuadcopters_SiFi/FCS/Logging ==
  motorCmds : Inport
  posRef : Inport  Port=2
  states_estim : Inport  Port=3  OutDataTypeStr=Bus: statesEstim_t  BusOutputAsStruct=on
  ReferenceValueServerBus : Inport  Port=4  OutDataTypeStr=Bus: CommandBus  BusOutputAsStruct=on
  Sensors : Inport  Port=5  OutDataTypeStr=Bus: SensorsBus
  sensordata_datin : Inport  Port=6  OutDataTypeStr=Bus: sensordata_t
  Bus Selector1 : BusSelector  OutputSignals=usePosVIS_flag,opticalFlow_data,posVIS_data
  Bus Selector2 : BusSelector  OutputSignals=ddx,ddy,ddz,p,q,r,altitude_sonar,prs,vbat_V,vbat_percentage
  Bus Selector3 : BusSelector  OutputSignals=controlModePosVSOrient,pos_ref,takeoff_flag,orient_ref,live_time_ticks
  Bus Selector4 : BusSelector  OutputSignals=X,Y,Z,yaw,pitch,roll,dx,dy,dz,p,q,r
  Bus Selector5 : BusSelector  OutputSignals=VisionSensors,SensorCalibration
  Data Type Conversion{,1..21} (22 alike) : DataTypeConversion  OutDataTypeStr=double
  FAULT_Data Type Conversion{,1..21} (22 alike) : F_Line_block/Subsystem
  Mux : Mux  Inputs=3
  FAULT_Mux{,1..3} (4 alike) : F_Line_block/Subsystem
  FAULT_Mux_2 : F_Line_block/Subsystem
  FAULT_Mux_3 : F_Line_block/Subsystem
  Mux1 : Mux  Inputs=5
  FAULT_Mux1_{2..5} (4 alike) : F_Line_block/Subsystem
  Mux2 : Mux  Inputs=12
  FAULT_Mux2_{2..12} (11 alike) : F_Line_block/Subsystem
  Mux3 : Mux  Inputs=10
  FAULT_Mux3_{2..10} (9 alike) : F_Line_block/Subsystem
  To Workspace : ToWorkspace  VariableName=motor  SaveFormat=Structure With Time  SampleTime=-1
  FAULT_motor : F_Line_block/Subsystem
  To Workspace1 : ToWorkspace  VariableName=posref  SaveFormat=Structure With Time  SampleTime=-1
  FAULT_posref : F_Line_block/Subsystem
  To Workspace2 : ToWorkspace  VariableName=estim  SaveFormat=Structure With Time  SampleTime=-1
  FAULT_estim : F_Line_block/Subsystem
  To Workspace3 : ToWorkspace  VariableName=cmd  SaveFormat=Structure With Time  SampleTime=-1
  FAULT_cmd : F_Line_block/Subsystem
  To Workspace4 : ToWorkspace  VariableName=optical  SaveFormat=Structure With Time  SampleTime=-1
  FAULT_optical : F_Line_block/Subsystem
  To Workspace5 : ToWorkspace  VariableName=calib  SaveFormat=Structure With Time  SampleTime=-1
  FAULT_calib : F_Line_block/Subsystem
  To Workspace6 : ToWorkspace  VariableName=sensor  SaveFormat=Structure With Time  SampleTime=-1
  FAULT_sensor : F_Line_block/Subsystem
  wires:
  Bus Selector3/1 -> FAULT_Data Type Conversion3/1  "<controlModePosVSOrient>"
  FAULT_Data Type Conversion3/1 -> Data Type Conversion3/1
  Bus Selector3/3 -> FAULT_Data Type Conversion7/1  "<takeoff_flag>"
  FAULT_Data Type Conversion7/1 -> Data Type Conversion7/1
  Bus Selector3/4 -> FAULT_Data Type Conversion8/1  "<orient_ref>"
  FAULT_Data Type Conversion8/1 -> Data Type Conversion8/1
  Bus Selector3/5 -> FAULT_Data Type Conversion9/1  "<live_time_ticks>"
  FAULT_Data Type Conversion9/1 -> Data Type Conversion9/1
  ReferenceValueServerBus/1 -> Bus Selector3/1
  Bus Selector3/2 -> FAULT_Data Type Conversion6/1  "<pos_ref>"
  FAULT_Data Type Conversion6/1 -> Data Type Conversion6/1
  sensordata_datin/1 -> Bus Selector2/1
  Bus Selector2/1 -> FAULT_Data Type Conversion/1  "<ddx>"
  FAULT_Data Type Conversion/1 -> Data Type Conversion/1
  Sensors/1 -> Bus Selector5/1
  Bus Selector1/1 -> FAULT_Data Type Conversion11/1  "<usePosVIS_flag>"
  FAULT_Data Type Conversion11/1 -> Data Type Conversion11/1
  Bus Selector1/2 -> FAULT_Data Type Conversion10/1  "<opticalFlow_data>"
  FAULT_Data Type Conversion10/1 -> Data Type Conversion10/1
  Bus Selector1/3 -> FAULT_Data Type Conversion2/1  "<posVIS_data>"
  FAULT_Data Type Conversion2/1 -> Data Type Conversion2/1
  Data Type Conversion1/1 -> To Workspace5/1
  Bus Selector5/2 -> FAULT_Data Type Conversion1/1  "<SensorCalibration>"
  FAULT_Data Type Conversion1/1 -> Data Type Conversion1/1
  Mux/1 -> To Workspace4/1
  Data Type Conversion4/1 -> To Workspace2/1
  motorCmds/1 -> FAULT_Data Type Conversion5/1
  FAULT_Data Type Conversion5/1 -> Data Type Conversion5/1
  Data Type Conversion5/1 -> To Workspace/1
  Mux1/1 -> To Workspace3/1
  states_estim/1 -> Bus Selector4/1
  Mux2/1 -> FAULT_Data Type Conversion4/1
  FAULT_Data Type Conversion4/1 -> Data Type Conversion4/1
  Bus Selector4/4 -> FAULT_Mux2_4/1  "<yaw>"
  FAULT_Mux2_4/1 -> Mux2/4
  Bus Selector4/6 -> ?  "<roll>"
  FAULT_Mux2_4/1 -> Mux2/4
  Bus Selector4/5 -> FAULT_Mux2_5/1  "<pitch>"
  FAULT_Mux2_5/1 -> Mux2/5
  Bus Selector4/9 -> ?  "<dz>"
  FAULT_Mux2_5/1 -> Mux2/5
  Bus Selector4/7 -> ?  "<dx>"
  FAULT_Mux2_5/1 -> Mux2/5
  Bus Selector4/8 -> ?  "<dy>"
  FAULT_Mux2_5/1 -> Mux2/5
  Bus Selector4/10 -> FAULT_Mux2/10  "<p>"
  FAULT_Mux2/1 -> Mux2/1
  Bus Selector4/12 -> FAULT_Mux2/12  "<r>"
  FAULT_Mux2/1 -> Mux2/1
  Bus Selector4/2 -> FAULT_Mux2_2/1  "<Y>"
  FAULT_Mux2_2/1 -> Mux2/2
  Bus Selector4/11 -> FAULT_Mux2/11  "<q>"
  FAULT_Mux2/1 -> Mux2/1
  Bus Selector4/3 -> FAULT_Mux2_3/1  "<Z>"
  FAULT_Mux2_3/1 -> Mux2/3
  Bus Selector4/1 -> FAULT_Mux2/1  "<X>"
  FAULT_Mux2/1 -> Mux2/1
  Data Type Conversion3/1 -> FAULT_Mux1/1
  FAULT_Mux1/1 -> Mux1/1
  Data Type Conversion6/1 -> FAULT_Mux1_2/1
  FAULT_Mux1_2/1 -> Mux1/2
  Data Type Conversion7/1 -> FAULT_Mux1_3/1
  FAULT_Mux1_3/1 -> Mux1/3
  Data Type Conversion8/1 -> FAULT_Mux1_4/1
  FAULT_Mux1_4/1 -> Mux1/4
  Data Type Conversion9/1 -> FAULT_Mux1_5/1
  FAULT_Mux1_5/1 -> Mux1/5
  Data Type Conversion2/1 -> FAULT_Mux_3/1
  FAULT_Mux_3/1 -> Mux/3
  Data Type Conversion10/1 -> FAULT_Mux_2/1
  FAULT_Mux_2/1 -> Mux/2
  Data Type Conversion11/1 -> FAULT_Mux/1
  FAULT_Mux/1 -> Mux/1
  posRef/1 -> FAULT_Data Type Conversion12/1
  FAULT_Data Type Conversion12/1 -> Data Type Conversion12/1
  Data Type Conversion12/1 -> To Workspace1/1
  Bus Selector2/2 -> FAULT_Data Type Conversion13/1  "<ddy>"
  FAULT_Data Type Conversion13/1 -> Data Type Conversion13/1
  Bus Selector2/3 -> FAULT_Data Type Conversion14/1  "<ddz>"
  FAULT_Data Type Conversion14/1 -> Data Type Conversion14/1
  Bus Selector2/4 -> FAULT_Data Type Conversion15/1  "<p>"
  FAULT_Data Type Conversion15/1 -> Data Type Conversion15/1
  Bus Selector2/5 -> FAULT_Data Type Conversion16/1  "<q>"
  FAULT_Data Type Conversion16/1 -> Data Type Conversion16/1
  Bus Selector2/6 -> FAULT_Data Type Conversion17/1  "<r>"
  FAULT_Data Type Conversion17/1 -> Data Type Conversion17/1
  Bus Selector2/7 -> FAULT_Data Type Conversion18/1  "<altitude_sonar>"
  FAULT_Data Type Conversion18/1 -> Data Type Conversion18/1
  Bus Selector2/8 -> FAULT_Data Type Conversion19/1  "<prs>"
  FAULT_Data Type Conversion19/1 -> Data Type Conversion19/1
  Bus Selector2/9 -> FAULT_Data Type Conversion20/1  "<vbat_V>"
  FAULT_Data Type Conversion20/1 -> Data Type Conversion20/1
  Bus Selector2/10 -> FAULT_Data Type Conversion21/1  "<vbat_percentage>"
  FAULT_Data Type Conversion21/1 -> Data Type Conversion21/1
  Data Type Conversion/1 -> FAULT_Mux3/1
  FAULT_Mux3/1 -> Mux3/1
  Data Type Conversion13/1 -> FAULT_Mux3_2/1
  FAULT_Mux3_2/1 -> Mux3/2
  Data Type Conversion14/1 -> FAULT_Mux3_3/1
  FAULT_Mux3_3/1 -> Mux3/3
  Data Type Conversion15/1 -> FAULT_Mux3_4/1
  FAULT_Mux3_4/1 -> Mux3/4
  Data Type Conversion16/1 -> FAULT_Mux3_5/1
  FAULT_Mux3_5/1 -> Mux3/5
  Data Type Conversion17/1 -> ?
  FAULT_Mux3_5/1 -> Mux3/5
  Data Type Conversion18/1 -> ?
  FAULT_Mux3_5/1 -> Mux3/5
  Data Type Conversion19/1 -> ?
  FAULT_Mux3_5/1 -> Mux3/5
  Data Type Conversion20/1 -> ?
  FAULT_Mux3_5/1 -> Mux3/5
  Data Type Conversion21/1 -> FAULT_Mux3/10
  FAULT_Mux3/1 -> Mux3/1
  Mux3/1 -> To Workspace6/1
  Bus Selector5/1 -> Bus Selector1/1  "<VisionSensors>"

== system asbQuadcopters_SiFi/FCS/State Estimator ==
  note: Derived frrom the work by Sertac
      | Karaman and Fabian Riether
  controlModePosVSOrient_flagin : Inport  OutDataTypeStr=boolean
  sensor_data_in : Inport  Port=2
  usePosVIS_flagin : Inport  Port=3
  opticalFlow_datin : Inport  Port=4
  posVIS_datin : Inport  Port=5
  sensorCalibration_datin : Inport  Port=6
  Complementary Filter : Subsystem
  Delay1 : Delay  DelayLength=1  InitialCondition=0
  FAULT_Delay1 : F_Line_block/Subsystem
  Demux : Demux  Outputs=3
  FAULT_Demux{,1,3..4} (4 alike) : F_Line_block/Subsystem
  Demux1 : Demux  Outputs=3
  Demux3 : Demux  Outputs=2
  Demux4 : Demux  Outputs=2
  EstimatorAltitude : Subsystem
  EstimatorXYPosition : Subsystem
  SensorPreprocessing : Subsystem
  Terminator : Terminator
  Terminator1 : Terminator
  posVIS_datin1 : InportShadow  Port=5
  usePosVIS_flagin1 : InportShadow  Port=3
  Out Bus Element : Outport  PortName=states_estim  Element=X
  Out Bus Element1 : Outport  PortName=states_estim  Element=Y
  Out Bus Element2 : Outport  PortName=states_estim  Element=Z
  Out Bus Element3 : Outport  PortName=states_estim  Element=yaw
  Out Bus Element4 : Outport  PortName=states_estim  Element=pitch
  Out Bus Element5 : Outport  PortName=states_estim  Element=roll
  Out Bus Element6 : Outport  PortName=states_estim  Element=dx
  Out Bus Element7 : Outport  PortName=states_estim  Element=dy
  Out Bus Element8 : Outport  PortName=states_estim  Element=dz
  Out Bus Element9 : Outport  PortName=states_estim  Element=p
  Out Bus Element10 : Outport  PortName=states_estim  Element=q
  Out Bus Element11 : Outport  PortName=states_estim  Element=r
  wires:
  EstimatorXYPosition/2(dxy_estimout) -> Delay1/1, Demux3/1
  posVIS_datin/1 -> SensorPreprocessing/2(posVIS_datin)
  Demux1/3 -> Out Bus Element11/1  "r"
  Demux/3 -> Out Bus Element5/1  "roll"
  Demux4/2 -> Out Bus Element1/1  "Y"
  EstimatorXYPosition/1(XY_estimout) -> Demux4/1
  Complementary Filter/2(deuler_datout) -> Terminator1/1
  Complementary Filter/4(dorient_estimaout) -> Demux1/1
  SensorPreprocessing/3(validVIS_flagout) -> Complementary Filter/3(validVis)
  sensor_data_in/1 -> SensorPreprocessing/3(sensordata_datin)
  opticalFlow_datin/1 -> EstimatorXYPosition/1(opticalFlow_datin)
  Demux4/1 -> Out Bus Element/1  "X"
  SensorPreprocessing/1(sensorIMU_datout) -> Complementary Filter/1(sensorIMU), EstimatorAltitude/1(sensorIMU_datin), EstimatorXYPosition/5(sensorIMU_datin)
  SensorPreprocessing/5(prsDelta_datout) -> EstimatorAltitude/3(prsDelta_datin)
  Demux3/2 -> Out Bus Element7/1  "dy"
  SensorPreprocessing/2(yawVis_datout) -> Complementary Filter/2(yawVIS)
  SensorPreprocessing/4(altSonar_datout) -> EstimatorAltitude/2(altSonar_datin)
  usePosVIS_flagin/1 -> SensorPreprocessing/1(usePosVIS_flagin)
  EstimatorAltitude/1(dz_estimout) -> Out Bus Element8/1, EstimatorXYPosition/7(dz_estimin)  "dz"
  EstimatorAltitude/2(Z_estimout) -> Out Bus Element2/1, EstimatorXYPosition/6(Z_estimin)  "Z"
  Demux1/1 -> Out Bus Element9/1  "p"
  Demux3/1 -> Out Bus Element6/1  "dx"
  Complementary Filter/3(imu_abs) -> Terminator/1
  Demux/2 -> Out Bus Element4/1  "pitch"
  controlModePosVSOrient_flagin/1 -> EstimatorXYPosition/2(controlModePosVSOrient_flagin)
  Complementary Filter/1(orient_estimaout) -> EstimatorAltitude/5(orient_estimin), Demux/1, EstimatorXYPosition/8(orient_estimin)  "att"
  Demux/1 -> Out Bus Element3/1  "yaw"
  Delay1/1 -> EstimatorAltitude/4(dxy_estimin)
  Demux1/2 -> Out Bus Element10/1  "q"
  usePosVIS_flagin1/1 -> EstimatorXYPosition/3(usePosVIS_flagin)
  posVIS_datin1/1 -> EstimatorXYPosition/4(posVIS_datin)
  sensorCalibration_datin/1 -> SensorPreprocessing/4(sensorCalibration_datin)

== system asbQuadcopters_SiFi/FCS/controller ==
  In Bus Element1 : Inport  PortName=ReferenceValueServerBus  Element=controlModePosVSOrient
  In Bus Element : Inport  PortName=ReferenceValueServerBus  Element=pos_ref
  In Bus Element4 : Inport  PortName=ReferenceValueServerBus  Element=pos_ref
  In Bus Element5 : Inport  PortName=ReferenceValueServerBus  Element=pos_ref
  In Bus Element2 : Inport  PortName=ReferenceValueServerBus  Element=orient_ref
  In Bus Element6 : Inport  PortName=ReferenceValueServerBus  Element=orient_ref
  In Bus Element7 : Inport  PortName=ReferenceValueServerBus  Element=orient_ref
  In Bus Element3 : Inport  PortName=ReferenceValueServerBus  Element=takeoff_flag
  states_estim : Inport  Port=2
  Attitude : Subsystem
  ControlMixer : Subsystem
  Mux2 : Mux  Inputs=3
  Selector : Selector  InputPortWidth=3  IndexOptions=Index vector (dialog)  Indices=3  OutputSizes=1
  Selector1 : Selector  InputPortWidth=3  IndexOptions=Index vector (dialog)  Indices=[1 2]  OutputSizes=1
  Selector2 : Selector  InputPortWidth=3  IndexOptions=Index vector (dialog)  Indices=[2 3]  OutputSizes=1
  Selector3 : Selector  InputPortWidth=3  IndexOptions=Index vector (dialog)  Indices=1  OutputSizes=1
  Switch_refAtt : Switch  Criteria=u2 > Threshold
  XY-to-reference-orientation : Subsystem
  Yaw : Subsystem
  gravity feedforward/equilibrium thrust : Subsystem
  states_estim1 : InportShadow  Port=2
  states_estim2 : InportShadow  Port=2
  states_estim3 : InportShadow  Port=2
  thrustsToMotorCommands : Subsystem
  motors_refout : Outport
  pose_refout : Outport  Port=2
  wires:
  thrustsToMotorCommands/1(motors_cmdout) -> motors_refout/1
  In Bus Element1/1 -> Switch_refAtt/2
  XY-to-reference-orientation/1(pitch_roll_cmd) -> Switch_refAtt/1
  In Bus Element2/1 -> Selector3/1
  In Bus Element/1 -> Selector1/1
  Selector3/1 -> Yaw/1(yaw_ref)
  Selector1/1 -> XY-to-reference-orientation/1(posXY)  "pos"
  ControlMixer/1(thrusts_refout) -> thrustsToMotorCommands/1(thrusts_refin)
  In Bus Element3/1 -> gravity feedforward/equilibrium thrust/3(takeoff_flag)
  states_estim/1 -> Yaw/2(states_estim)
  Switch_refAtt/1 -> Attitude/1(refAttitude), Mux2/3
  Yaw/1(yaw) -> XY-to-reference-orientation/3(yaw)
  gravity feedforward/equilibrium thrust/1(altitude_cmd) -> ControlMixer/4(totalThrust)
  Mux2/1 -> pose_refout/1
  Attitude/1(tau_pitch) -> ControlMixer/1(tau_pitch)
  Attitude/2(tau_roll) -> ControlMixer/2(tau_roll)
  Yaw/2(tau_yaw) -> ControlMixer/3(tau_yaw)
  states_estim1/1 -> gravity feedforward/equilibrium thrust/1(states_estim)
  states_estim2/1 -> Attitude/2(states_estim)
  states_estim3/1 -> XY-to-reference-orientation/2(states_estim)
  In Bus Element4/1 -> Mux2/1
  Selector/1 -> gravity feedforward/equilibrium thrust/2(PosZ)
  In Bus Element5/1 -> Selector/1
  In Bus Element6/1 -> Selector2/1
  Selector2/1 -> Switch_refAtt/3
  In Bus Element7/1 -> Mux2/2

== system asbQuadcopters_SiFi/FCS/sensordata_group ==
  HAL_acc_SI : Inport  OutDataTypeStr=Bus: HAL_acc_SI_t
  HAL_gyro_SI : Inport  Port=2  OutDataTypeStr=Bus: HAL_gyro_SI_t
  HAL_ultrasound_SI : Inport  Port=3  OutDataTypeStr=Bus: HAL_ultrasound_SI_t
  HAL_pressure_SI : Inport  Port=4  OutDataTypeStr=Bus: HAL_pressure_SI_t
  HAL_vbat_SI : Inport  Port=5  OutDataTypeStr=Bus: HAL_vbat_SI_t
  Bus Selector1 : BusSelector  OutputSignals=vbat_V,vbat_percentage
  Bus Selector3 : BusSelector  OutputSignals=x,y,z
  Bus Selector4 : BusSelector  OutputSignals=x,y,z
  Bus Selector5 : BusSelector  OutputSignals=altitude
  Bus Selector6 : BusSelector  OutputSignals=pressure
  Out Bus Element : Outport  PortName=sensordata_datin  Element=ddx
  Out Bus Element1 : Outport  PortName=sensordata_datin  Element=ddy
  Out Bus Element2 : Outport  PortName=sensordata_datin  Element=ddz
  Out Bus Element3 : Outport  PortName=sensordata_datin  Element=p
  Out Bus Element4 : Outport  PortName=sensordata_datin  Element=q
  Out Bus Element5 : Outport  PortName=sensordata_datin  Element=r
  Out Bus Element6 : Outport  PortName=sensordata_datin  Element=altitude_sonar
  Out Bus Element7 : Outport  PortName=sensordata_datin  Element=prs
  Out Bus Element8 : Outport  PortName=sensordata_datin  Element=vbat_V
  Out Bus Element9 : Outport  PortName=sensordata_datin  Element=vbat_percentage
  wires:
  HAL_gyro_SI/1 -> Bus Selector4/1
  HAL_acc_SI/1 -> Bus Selector3/1
  HAL_pressure_SI/1 -> Bus Selector6/1
  HAL_ultrasound_SI/1 -> Bus Selector5/1
  Bus Selector4/1 -> Out Bus Element3/1  "<x>"
  Bus Selector3/3 -> Out Bus Element2/1  "<z>"
  Bus Selector4/3 -> Out Bus Element5/1  "<z>"
  Bus Selector5/1 -> Out Bus Element6/1  "<altitude>"
  Bus Selector6/1 -> Out Bus Element7/1  "<pressure>"
  Bus Selector4/2 -> Out Bus Element4/1  "<y>"
  Bus Selector3/1 -> Out Bus Element/1  "<x>"
  Bus Selector3/2 -> Out Bus Element1/1  "<y>"
  Bus Selector1/1 -> Out Bus Element8/1  "<vbat_V>"
  HAL_vbat_SI/1 -> Bus Selector1/1
  Bus Selector1/2 -> Out Bus Element9/1  "<vbat_percentage>"

== system asbQuadcopters_SiFi/Sensor/Sensor System ==
  States : Inport
  Environment : Inport  Port=2
  Camera : Subsystem
  IMU_Pressure : Subsystem
  Rate Transition1 : RateTransition  OutPortSampleTime=Ts
  Rate Transition2 : RateTransition  OutPortSampleTime=Ts
  opticalFlow_data : Outport
  sensordata_data : Outport  Port=2  OutDataTypeStr=Bus: HAL_acquisition_t
  wires:
  Rate Transition2/1 -> sensordata_data/1
  Camera/1(opticalFlow_datout) -> Rate Transition1/1
  Environment/1 -> IMU_Pressure/2(Environment)
  IMU_Pressure/1(sensordata_datout) -> Rate Transition2/1
  States/1 -> IMU_Pressure/1(States), Camera/1(states)
  Rate Transition1/1 -> opticalFlow_data/1

== system asbQuadcopters_SiFi/Visualization/Extract Flight Instruments ==
  Actuators : Inport
  States : Inport  Port=2
  Altitude [ft] : aerolibconvert2/Length Conversion  IU=m  OU=ft
  Altitude [m] : Selector  InputPortWidth=3  IndexOptions=Index vector (dialog)  Indices=[3]  OutputSizes=1
  Bus Selector : BusSelector  OutputSignals=LLA,Euler,V_ned,V_body,X_ned
  Deg from North : Bias  Bias=Vehicle.PositionOnEarth.FlatEarthToLLA.xAxis
  Demux : Demux  Outputs=3
  Demux1 : Demux
  Display{,1..8} (9 alike) : Display
  Euler [deg] : aerolibconvert2/Angle Conversion  IU=rad  OU=deg
  Floor contact : simulink/Model Verification/Check Static  Lower Bound  Description=init.posLLA(3) <= u  min=init.posLLA(3)  min_included=on  enabled=on  stopWhenAssertionFail=on  export=off  icon=graphic
      settings: SourceProductName=Simulink
  Gain : Gain  Gain=-1/1000
  Gain1 : Gain  Gain=100/Vehicle.Motor.maxLimit*[1 -1 1 -1]
  Math Function : Math  Operator=square  SaturateOnIntegerOverflow=on
  Mux : Mux  Inputs=2
  Sqrt : Sqrt  SaturateOnIntegerOverflow=on
  Sum of Elements : Sum  Inputs=+
  V : aerolibconvert2/Velocity Conversion  IU=m/s  OU=kts
  Vd [ft/min] : aerolibconvert2/Velocity Conversion  IU=m/s  OU=ft/min
  Vd [m/s] : Selector  InputPortWidth=3  IndexOptions=Index vector (dialog)  Indices=[3]  OutputSizes=1
  XY : Outport
  Actuator : Outport  Port=2
  wires:
  Bus Selector/1 -> Altitude [m]/1  "<LLA>"
  Altitude [m]/1 -> Floor contact/1, Altitude [ft]/1
  States/1 -> Bus Selector/1
  Altitude [ft]/1 -> Display/1
  Bus Selector/2 -> Euler [deg]/1  "<Euler>"
  Euler [deg]/1 -> Demux/1
  Demux/1 -> Mux/1
  Demux/2 -> Mux/2
  Mux/1 -> Display1/1
  Deg from North/1 -> Display2/1
  Bus Selector/3 -> Vd [m/s]/1  "<V_ned>"
  Vd [m/s]/1 -> Vd [ft/min]/1
  Vd [ft/min]/1 -> Gain/1
  Gain/1 -> Display3/1
  Math Function/1 -> Sum of Elements/1
  Sum of Elements/1 -> Sqrt/1
  Bus Selector/4 -> Math Function/1  "<V_body>"
  Sqrt/1 -> V/1
  V/1 -> Display4/1
  Gain1/1 -> Demux1/1
  Demux1/1 -> Display5/1
  Demux1/2 -> Display6/1
  Demux1/3 -> Display7/1
  Demux1/4 -> Display8/1
  Actuators/1 -> Actuator/1, Gain1/1
  Demux/3 -> Deg from North/1
  Bus Selector/5 -> XY/1  "<X_ned>"

== system asbQuadcopters_SiFi/Airframe/AC model/Applied Force Calculation ==
  gravity force : Inport  Unit=N
  Aerodynamic Forces : Inport  Port=2  Unit=N
  Motor Forces : Inport  Port=3  Unit=N
  Add1 : Sum  Inputs=+++
  FAULT_Add1 : F_Line_block/Subsystem
  FAULT_Add1_2 : F_Line_block/Subsystem
  FAULT_Add1_3 : F_Line_block/Subsystem
  Signal Specification : SignalSpecification  Dimensions=3
  FAULT_Signal Specification : F_Line_block/Subsystem
  External Forces : Outport  Unit=N
  FAULT_External Forces : F_Line_block/Subsystem
  wires:
  Add1/1 -> FAULT_Signal Specification/1
  FAULT_Signal Specification/1 -> Signal Specification/1
  Motor Forces/1 -> FAULT_Add1_3/1  "Motor Thrust"
  FAULT_Add1_3/1 -> Add1/3
  Aerodynamic Forces/1 -> FAULT_Add1_2/1
  FAULT_Add1_2/1 -> Add1/2
  gravity force/1 -> FAULT_Add1/1
  FAULT_Add1/1 -> Add1/1
  Signal Specification/1 -> FAULT_External Forces/1
  FAULT_External Forces/1 -> External Forces/1

== system asbQuadcopters_SiFi/Airframe/AC model/Drag Calculation ==
  Density : Inport  Unit=kg/m^3
  Vb : Inport  Port=2  Unit=m/second
  Drag Calc : Subsystem
  Gain3 : Gain  Gain=-1
  FAULT_Gain3 : F_Line_block/Subsystem
  Product : Product  RndMeth=Zero
  FAULT_Product : F_Line_block/Subsystem
  FAULT_Product_2 : F_Line_block/Subsystem
  Sign : Signum  ZeroCross=off
  FAULT_Sign : F_Line_block/Subsystem
  Drag : Outport  Unit=N
  FAULT_Drag : F_Line_block/Subsystem
  wires:
  Density/1 -> Drag Calc/1(Density)
  Sign/1 -> FAULT_Gain3/1
  FAULT_Gain3/1 -> Gain3/1
  Drag Calc/1(drag) -> FAULT_Product/1
  FAULT_Product/1 -> Product/1
  Gain3/1 -> FAULT_Product_2/1
  FAULT_Product_2/1 -> Product/2
  Product/1 -> FAULT_Drag/1  "xDrag"
  FAULT_Drag/1 -> Drag/1
  Vb/1 -> FAULT_Sign/1, Drag Calc/2(vel)
  FAULT_Sign/1 -> Sign/1
  ?FAULT_Mux1_2/1 -> ?Mux1/2
